simulink model "commtimrecresample"  (Simulink 7.2)
settings: Solver=ode45  StartTime=0.0  StopTime=5e-3  MaxStep=1/(10*D*Fsymbol)  RelTol=1e-3
PreLoadFcn:
  | Fsymbol=1e6;
  | D=8;  % decimation / interpolation
  | Fdelay = 5;  % rrc filter delay
  | Alpha = 0.25;  % excess BW
  | rrc_coef=rcosine(1,D,'fir/sqrt',Alpha,Fdelay);
  | rrc_coef=rrc_coef/sum(rrc_coef);
  | Carrier_Freq = 21.4e6;
  | b3 = [1/6 -1/2  1/2 -1/6];
  | b2 = [1/2 -1    1/2  0];
  | b1 = [1/3  1/2 -1    1/6];
  | b0 = [0    1    0    0];
undefined symbols (not defined in the file or in its folder): dfilt, j, magnitude
libraries: dspsigops x29, simulink x12, dsparch4 x8, commsynccomp2 x3, dspbuff3 x2, commblksprivate x1, dspmlti4 x1, commsink2 x1
Description:
  | Timing Recovery using Fixed-Rate Resampling
CloseFcn:
  | clear Fsymbol D Fdelay Alpha rrc_coef Carrier_Freq b0 b1 b2 b3;
settings Model: Creator=The MathWorks Inc.  LastModifiedBy=user
settings SolverCC: InsertRTBMode=Auto  SignalSizeVariationType=Allow to vary during execution
settings DataIOCC: SaveOutput=off  SignalLogging=off  SaveTime=off
settings OptimizationCC: InitFltsAndDblsToZero=on  EfficientMapNaN2IntZero=off
settings DebuggingCC: SaveWithParameterizedLinksMsg=none  SignalResolutionControl=TryResolveAllWithWarning  MultiTaskDSMMsg=warning  MultiTaskCondExecSysMsg=none  SigSpecEnsureSampleTimeMsg=none  StrictBusMsg=None
settings RTWCC: IncludeERTFirstTime=on
settings GRTTargetCC: TargetFcnLib=ansi_tfl_tmw.mat

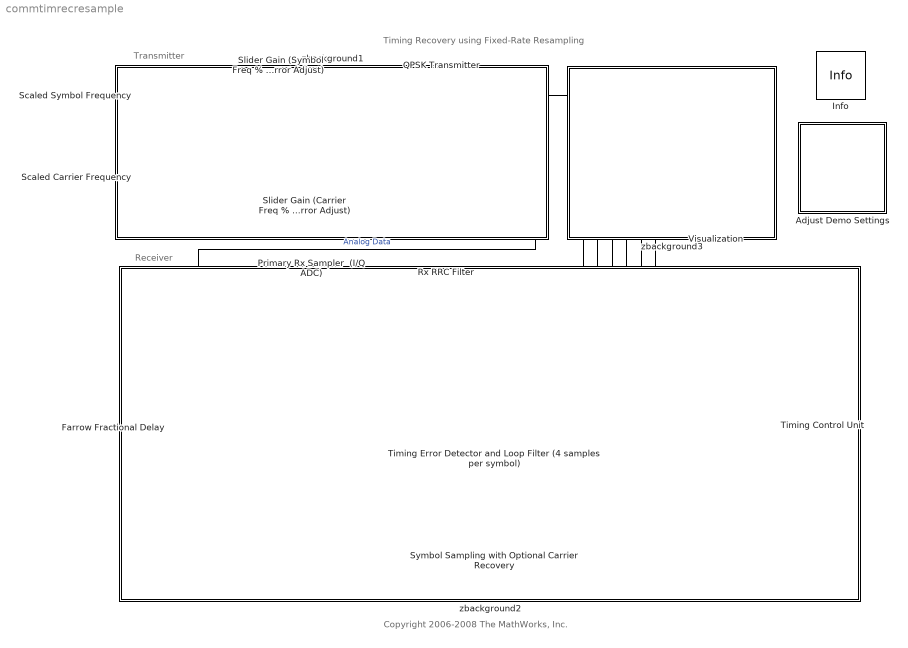
== system commtimrecresample ==
  note: Timing Recovery using Fixed-Rate Resampling
  note: Transmitter
  note: Receiver
  note: Copyright 2006-2008 The MathWorks, Inc.
  Adjust Demo Settings : Subsystem  mask(Timing Recovery Demo Settings){enableCarrierRec=on, enableTCU=on}
      mask prompts: enableCarrierRec "Enable carrier recovery"; enableTCU "Enable timing control"
      mask help:
      | Adjust these demo parameter settings to change the characteristics of the timing recovery (receiver) subsystem.  These settings may be changed while the demo is running.
      |
      | Note that you can also change the slider gain values for Symbol Frequency Percent Error and Carrier Frequency Percent Error while the demo is running.
      mask init:
      | set_param([bdroot(gcb) '/Symbol Sampling with Optional Carrier Recovery/Carrier_Rec_ON'],'Value',num2str(enableCarrierRec));
      | set_param([bdroot(gcb) '/Timing Control Unit/TCU_ON'],'Value',num2str(enableTCU));
      mask Help: helpview(commdhelp);
      mask Display: disp('Timing\nRecovery\nDemo\nSettings');
  "Farrow Fractional Delay " : Subsystem
  Info : commblksprivate/Info  SystemSampleTime=-1
  Primary Rx Sampler  (I/Q ADC) : ZeroOrderHold  SampleTime=1/(D*Fsymbol)
  QPSK Transmitter : Subsystem
  Rx RRC Filter : dspmlti4/FIR Decimation  DialogController=dspdialog.FIRDecimation  DialogControllerArgs=DataTag5  h=rrc_coef  D=2  filtStruct=Direct form  framing=Maintain input frame size  outputBufInitCond=0  roundingMode=Floor  overflowMode=off  FilterSource=Specify via dialog  FilterObject=Hm_firdecim
  Scaled Carrier Frequency : Constant  Value=Carrier_Freq / 100  OutDataType=sfix(16)  OutScaling=2^0
  Scaled Symbol Frequency : Constant  Value=(D*Fsymbol) / 100  OutDataType=sfix(16)  OutScaling=2^0
  Slider Gain (Carrier Freq % Error Adjust) : simulink/Math Operations/Slider Gain  SystemSampleTime=-1  low=-0.2  gain=-0.02  high=0.2
  Slider Gain (Symbol Freq % Error Adjust) : simulink/Math Operations/Slider Gain  SystemSampleTime=-1  low=-0.2  gain=0.05  high=0.2
  Symbol Sampling with Optional Carrier Recovery : Subsystem
  Timing Control Unit : Subsystem
  Timing Error Detector and Loop Filter (4 samples per symbol) : Subsystem
  Visualization : Subsystem
  zbackground1 : Subsystem
      mask Display: disp('')
  zbackground2 : Subsystem
      mask Display: disp('')
  zbackground3 : Subsystem
      mask Display: disp('')
  wires:
  Scaled Symbol Frequency/1 -> Slider Gain (Symbol Freq % Error Adjust)/1
  Slider Gain (Symbol Freq % Error Adjust)/1 -> QPSK Transmitter/1(Tx Sym Err)
  Slider Gain (Carrier Freq % Error Adjust)/1 -> QPSK Transmitter/2(Tx Car Err)
  Scaled Carrier Frequency/1 -> Slider Gain (Carrier Freq % Error Adjust)/1
  QPSK Transmitter/1(Tx Sym Clk) -> Visualization/1(Tx Sym Clk)
  QPSK Transmitter/2(Tx Data) -> Primary Rx Sampler  (I/Q ADC)/1  "Analog Data"
  "Farrow Fractional Delay "/1(X(n-(1-u))) -> Timing Error Detector and Loop Filter (4 samples per symbol)/2(I/Q In), Symbol Sampling with Optional Carrier Recovery/2(Data)
  Primary Rx Sampler  (I/Q ADC)/1 -> Rx RRC Filter/1
  Rx RRC Filter/1 -> "Farrow Fractional Delay "/1(X(n))
  Timing Control Unit/1(Symbol Clk) -> Timing Error Detector and Loop Filter (4 samples per symbol)/1(Symbol Clk), Symbol Sampling with Optional Carrier Recovery/1(Symbol Clk), Visualization/2(Rx Rec Sym Clk)
  Timing Control Unit/2(Delay Ctrl) -> "Farrow Fractional Delay "/2(u), Visualization/7(Frac Dly Ctrl)
  Timing Error Detector and Loop Filter (4 samples per symbol)/2(Timing Ctrl) -> Timing Control Unit/1(Ctrl In), Visualization/4(TCU Ctrl)
  Timing Error Detector and Loop Filter (4 samples per symbol)/1(Timing Err) -> Visualization/3(Timing Err)
  Symbol Sampling with Optional Carrier Recovery/1(Delayed Clk) -> Visualization/5(Delayed Clk)
  Symbol Sampling with Optional Carrier Recovery/2(Symbol) -> Visualization/6(Rx Symbol)

== system commtimrecresample/Adjust Demo Settings ==

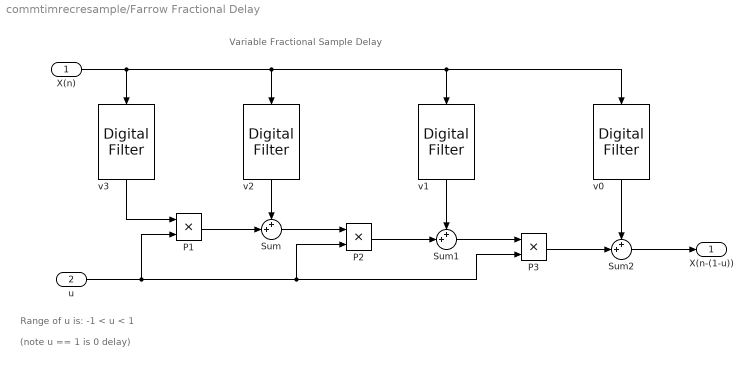
== system commtimrecresample/Farrow Fractional Delay  ==
  note: Range of u is: -1 < u < 1
  note: Variable Fractional Sample Delay
  note: (note u == 1 is 0 delay)
  X(n) : Inport  OutDataType=sfix(16)  OutScaling=2^0
  u : Inport  Port=2  OutDataType=sfix(16)  OutScaling=2^0
  P1 : Product  OutDataType=sfix(16)  OutScaling=2^0  SaturateOnIntegerOverflow=on  OutDataTypeStr=Inherit: Same as first input
  P2 : Product  OutDataType=sfix(16)  OutScaling=2^0  SaturateOnIntegerOverflow=on  OutDataTypeStr=Inherit: Same as first input
  P3 : Product  OutDataType=sfix(16)  OutScaling=2^0  SaturateOnIntegerOverflow=on  OutDataTypeStr=Inherit: Same as first input
  Sum : Sum  Inputs=++|  OutDataType=sfix(16)  OutScaling=2^0  SaturateOnIntegerOverflow=on
  Sum1 : Sum  Inputs=++|  OutDataType=sfix(16)  OutScaling=2^0  SaturateOnIntegerOverflow=on
  Sum2 : Sum  Inputs=++|  OutDataType=sfix(16)  OutScaling=2^0  SaturateOnIntegerOverflow=on
  v0 : dsparch4/Digital Filter  Orientation=down  DialogController=dspdialog.DigitalFilter  DialogControllerArgs=DataTag0  TypePopup=FIR (all zeros)  IIRFiltStruct=Direct form II transposed  AllPoleFiltStruct=Direct form  FIRFiltStruct=Direct form  CoeffSource=Specify via dialog  NumCoeffs=b0  DenCoeffs=[1 0.1]  BiQuadCoeffs=[1 0.3 0.4 1 0.1 0.2]  LatticeCoeffs=[0.2 0.4]  denIgnore=on  FiltPerSampPopup=One filter per frame  IC=0  ICnum=0  ICden=0  roundingMode=Floor  overflowMode=off  ScaleValues=1  scaleValueFracLength=14  stageInFracLength=15  stageOutFracLength=15  FilterSource=Specify via dialog  dfiltObjectName=dfilt.dffir([1 2 1])
  v1 : dsparch4/Digital Filter  Orientation=down  DialogController=dspdialog.DigitalFilter  DialogControllerArgs=DataTag1  TypePopup=FIR (all zeros)  IIRFiltStruct=Direct form II transposed  AllPoleFiltStruct=Direct form  FIRFiltStruct=Direct form  CoeffSource=Specify via dialog  NumCoeffs=b1  DenCoeffs=[1 0.1]  BiQuadCoeffs=[1 0.3 0.4 1 0.1 0.2]  LatticeCoeffs=[0.2 0.4]  denIgnore=on  FiltPerSampPopup=One filter per frame  IC=0  ICnum=0  ICden=0  roundingMode=Floor  overflowMode=off  ScaleValues=1  scaleValueFracLength=14  stageInFracLength=15  stageOutFracLength=15  FilterSource=Specify via dialog  dfiltObjectName=dfilt.dffir([1 2 1])
  v2 : dsparch4/Digital Filter  Orientation=down  DialogController=dspdialog.DigitalFilter  DialogControllerArgs=DataTag2  TypePopup=FIR (all zeros)  IIRFiltStruct=Direct form II transposed  AllPoleFiltStruct=Direct form  FIRFiltStruct=Direct form  CoeffSource=Specify via dialog  NumCoeffs=b2  DenCoeffs=[1 0.1]  BiQuadCoeffs=[1 0.3 0.4 1 0.1 0.2]  LatticeCoeffs=[0.2 0.4]  denIgnore=on  FiltPerSampPopup=One filter per frame  IC=0  ICnum=0  ICden=0  roundingMode=Floor  overflowMode=off  ScaleValues=1  scaleValueFracLength=14  stageInFracLength=15  stageOutFracLength=15  FilterSource=Specify via dialog  dfiltObjectName=dfilt.dffir([1 2 1])
  v3 : dsparch4/Digital Filter  Orientation=down  DialogController=dspdialog.DigitalFilter  DialogControllerArgs=DataTag3  TypePopup=FIR (all zeros)  IIRFiltStruct=Direct form II transposed  AllPoleFiltStruct=Direct form  FIRFiltStruct=Direct form  CoeffSource=Specify via dialog  NumCoeffs=b3  DenCoeffs=[1 0.1]  BiQuadCoeffs=[1 0.3 0.4 1 0.1 0.2]  LatticeCoeffs=[0.2 0.4]  denIgnore=on  FiltPerSampPopup=One filter per frame  IC=0  ICnum=0  ICden=0  roundingMode=Floor  overflowMode=off  ScaleValues=1  scaleValueFracLength=14  stageInFracLength=15  stageOutFracLength=15  FilterSource=Specify via dialog  dfiltObjectName=dfilt.dffir([1 2 1])
  X(n-(1-u)) : Outport  OutDataType=sfix(16)  OutScaling=2^0
  wires:
  Sum2/1 -> X(n-(1-u))/1
  u/1 -> P3/2, P2/2, P1/2
  X(n)/1 -> v3/1, v2/1, v1/1, v0/1
  v0/1 -> Sum2/1
  v1/1 -> Sum1/1
  v2/1 -> Sum/1
  v3/1 -> P1/1
  P1/1 -> Sum/2
  Sum/1 -> P2/1
  P2/1 -> Sum1/2
  Sum1/1 -> P3/1
  P3/1 -> Sum2/2

== system commtimrecresample/QPSK Transmitter ==
  note: 1/Ts=D*Fsymbol
  Tx Sym Err : Inport  OutDataType=sfix(16)  OutScaling=2^0
  Tx Car Err : Inport  Port=2  OutDataType=sfix(16)  OutScaling=2^0
  Carrier Offset and Conversion to Continuous Time : Subsystem
  Variable Rate Symbol Generator : Subsystem  TreatAsAtomicUnit=on
  Voltage-Controlled Oscillator : commsynccomp2/Continuous-Time VCO  SystemSampleTime=-1  Ac=1  Fc=D*Fsymbol  Kc=1  Ph=pi
  Tx Sym Clk : Outport  OutDataType=sfix(16)  OutScaling=2^0
  Tx Data : Outport  Port=2  OutDataType=sfix(16)  OutScaling=2^0
  wires:
  Variable Rate Symbol Generator/1(RRC'd Symbols) -> Carrier Offset and Conversion to Continuous Time/1(Data)
  Voltage-Controlled Oscillator/1 -> Variable Rate Symbol Generator/Trigger
  Carrier Offset and Conversion to Continuous Time/1(I/Q Out) -> Tx Data/1  "Baseband Continuous-Time Data"
  Tx Car Err/1 -> Carrier Offset and Conversion to Continuous Time/2(Error)
  Tx Sym Err/1 -> Voltage-Controlled Oscillator/1
  Variable Rate Symbol Generator/2(Symbol Clk) -> Tx Sym Clk/1  "Symbol Clock"

== system commtimrecresample/Symbol Sampling with Optional Carrier Recovery ==
  note: Subsequent processing (demodulation, error correction, symbol to bit mapping, etc.)
      | may be placed inside the Symbol Sampler block.
  Symbol Clk : Inport  OutDataType=sfix(16)  OutScaling=2^0
  Data : Inport  Port=2  OutDataType=sfix(16)  OutScaling=2^0
  Carrier_Rec_ON : Constant  OutDataTypeMode=boolean  OutDataType=sfix(16)  OutScaling=2^0  OutDataTypeStr=boolean
  Delay : dspsigops/Delay  dly_unit=Samples  delay=2  ic_detail=off  dif_ic_for_ch=off  dif_ic_for_dly=off  ic=0  reset_popup=None
  Symbol Sampler : Subsystem  TreatAsAtomicUnit=on
  Delayed Clk : Outport  OutDataType=sfix(16)  OutScaling=2^0
  Symbol : Outport  Port=2  OutDataType=sfix(16)  OutScaling=2^0
  wires:
  Delay/1 -> Delayed Clk/1, Symbol Sampler/Enable
  Symbol Clk/1 -> Delay/1
  Data/1 -> Symbol Sampler/1(In1)
  Symbol Sampler/1(Out1) -> Symbol/1
  Carrier_Rec_ON/1 -> Symbol Sampler/2(Carrier Recovery ON)

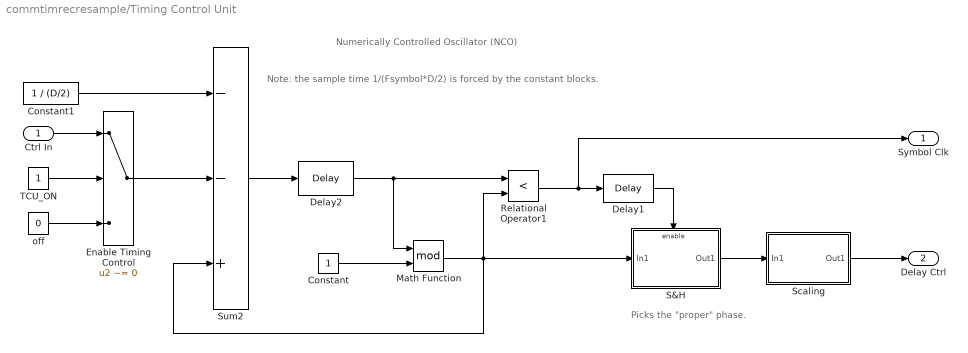
== system commtimrecresample/Timing Control Unit ==
  note: Note:  the sample time 1/(Fsymbol*D/2)
      | is forced by the constant blocks.
  note: Numerically Controlled Oscillator (NCO)
  note: Picks the "proper" phase.
  Ctrl In : Inport  OutDataType=sfix(16)  OutScaling=2^0
  Constant : Constant  OutDataType=sfix(16)  OutScaling=2^0  OutDataTypeStr=Inherit: Inherit via back propagation  SampleTime=1/(Fsymbol*D/2)
  Constant1 : Constant  Value=1 / (D/2)  OutDataType=sfix(16)  OutScaling=2^0  OutDataTypeStr=Inherit: Inherit via back propagation  SampleTime=1/(Fsymbol*D/2)
  Delay1 : dspsigops/Delay  dly_unit=Samples  delay=1  ic_detail=off  dif_ic_for_ch=off  dif_ic_for_dly=off  ic=0  reset_popup=None
  Delay2 : dspsigops/Delay  dly_unit=Samples  delay=1  ic_detail=on  dif_ic_for_ch=off  dif_ic_for_dly=off  ic=0  reset_popup=None
  Enable Timing Control : Switch  Criteria=u2 ~= 0
  Math Function : Math  Operator=mod  OutDataType=sfix(16)  OutScaling=2^0  SaturateOnIntegerOverflow=on
  Relational Operator1 : RelationalOperator  Operator=<  LogicOutDataTypeMode=boolean  LogicDataType=double(64)  OutDataTypeStr=boolean
  "S&H " : Subsystem  TreatAsAtomicUnit=on
  Scaling : Subsystem
  Sum2 : Sum  Inputs=--+  OutDataType=sfix(16)  OutScaling=2^0  SaturateOnIntegerOverflow=on  InputSameDT=on  OutDataTypeStr=Inherit: Same as first input
  TCU_ON : Constant  OutDataTypeMode=boolean  OutDataType=sfix(16)  OutScaling=2^0  OutDataTypeStr=boolean
  off : Constant  Value=0  OutDataType=sfix(16)  OutScaling=2^0
  Symbol Clk : Outport  OutDataType=sfix(16)  OutScaling=2^0
  Delay Ctrl : Outport  Port=2  OutDataType=sfix(16)  OutScaling=2^0
  wires:
  Delay2/1 -> Math Function/1, Relational Operator1/1
  Constant/1 -> Math Function/2
  Sum2/1 -> Delay2/1
  Constant1/1 -> Sum2/1
  Math Function/1 -> Sum2/3, Relational Operator1/2, "S&H "/1(In1)
  Relational Operator1/1 -> Delay1/1, Symbol Clk/1
  Delay1/1 -> "S&H "/Enable
  "S&H "/1(Out1) -> Scaling/1(In1)
  Scaling/1(Out1) -> Delay Ctrl/1
  TCU_ON/1 -> Enable Timing Control/2
  off/1 -> Enable Timing Control/3
  Ctrl In/1 -> Enable Timing Control/1
  Enable Timing Control/1 -> Sum2/2

== system commtimrecresample/Timing Error Detector and Loop Filter (4 samples per symbol) ==
  note: H. Meyer et. al. Digital Communications Receivers, chapter 5.4, pp 291
  Symbol Clk : Inport  OutDataType=sfix(16)  OutScaling=2^0
  I/Q In : Inport  Port=2  OutDataType=sfix(16)  OutScaling=2^0
  Mag Sq + Delays : Subsystem
  Timing Error Detector : Subsystem  TreatAsAtomicUnit=on
  Timing Err : Outport  OutDataType=sfix(16)  OutScaling=2^0
  Timing Ctrl : Outport  Port=2  OutDataType=sfix(16)  OutScaling=2^0
  wires:
  Mag Sq + Delays/1(MagSq(u[n-1])) -> Timing Error Detector/1(In1)
  Mag Sq + Delays/2(MagSq(u[n-3])) -> Timing Error Detector/2(In2)
  Mag Sq + Delays/3(MagSq(u[n-2])) -> Timing Error Detector/3(In3)
  Mag Sq + Delays/4(MagSq(u[n])) -> Timing Error Detector/4(In4)
  I/Q In/1 -> Mag Sq + Delays/1(In1)
  Timing Error Detector/1(Error) -> Timing Err/1
  Timing Error Detector/2(Cntrl) -> Timing Ctrl/1
  Symbol Clk/1 -> Timing Error Detector/Enable

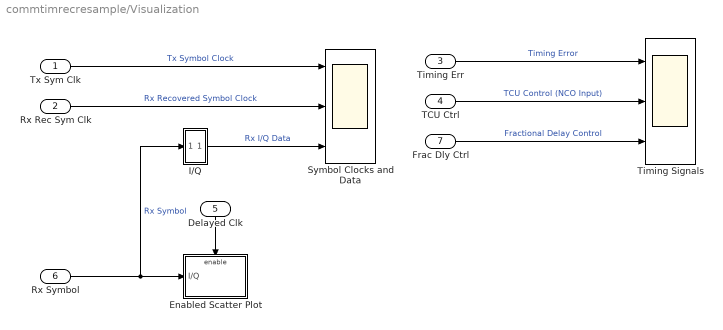
== system commtimrecresample/Visualization ==
  Tx Sym Clk : Inport  OutDataType=sfix(16)  OutScaling=2^0
  Rx Rec Sym Clk : Inport  Port=2  OutDataType=sfix(16)  OutScaling=2^0
  Timing Err : Inport  Port=3  OutDataType=sfix(16)  OutScaling=2^0
  TCU Ctrl : Inport  Port=4  OutDataType=sfix(16)  OutScaling=2^0
  Delayed Clk : Inport  Orientation=down  Port=5  OutDataType=sfix(16)  OutScaling=2^0
  Rx Symbol : Inport  Port=6  OutDataType=sfix(16)  OutScaling=2^0
  Frac Dly Ctrl : Inport  Port=7  OutDataType=sfix(16)  OutScaling=2^0
  Enabled Scatter Plot : Subsystem  TreatAsAtomicUnit=on
  I/Q : Subsystem
      mask Display: disp('')
  Symbol Clocks and Data : Scope  NumInputPorts=3
      settings: TimeRange=2e-006  YMin=-0.1~-0.1~-1.5  YMax=1.1~1.1~1.5
  Timing Signals : Scope  NumInputPorts=3
      settings: TimeRange=0.0002  YMin=-0.2~-0.001~-0.1  YMax=0.2~0.001~1.1  MaxDataPoints=50000
  wires:
  Rx Symbol/1 -> I/Q/1(cmplx), Enabled Scatter Plot/1(I/Q)  "Rx Symbol"
  I/Q/1(2x real) -> Symbol Clocks and Data/3  "Rx I/Q Data"
  Tx Sym Clk/1 -> Symbol Clocks and Data/1  "Tx Symbol Clock"
  Rx Rec Sym Clk/1 -> Symbol Clocks and Data/2  "Rx Recovered Symbol Clock"
  Timing Err/1 -> Timing Signals/1  "Timing Error"
  TCU Ctrl/1 -> Timing Signals/2  "TCU Control (NCO Input)"
  Frac Dly Ctrl/1 -> Timing Signals/3  "Fractional Delay Control"
  Delayed Clk/1 -> Enabled Scatter Plot/Enable

== system commtimrecresample/zbackground1 ==

== system commtimrecresample/zbackground2 ==

== system commtimrecresample/zbackground3 ==

== system commtimrecresample/QPSK Transmitter/Carrier Offset and Conversion to Continuous Time ==
  Data : Inport  OutDataType=sfix(16)  OutScaling=2^0
  Error : Inport  Port=2  OutDataType=sfix(16)  OutScaling=2^0
  Bessel LPF : Subsystem
  Product : Product  OutDataType=sfix(16)  OutScaling=2^0  RndMeth=Zero
  Real-Imag to Complex : RealImagToComplex
  Voltage-Controlled Oscillator : commsynccomp2/Continuous-Time VCO  SystemSampleTime=-1  Ac=1  Fc=0  Kc=1  Ph=0
  Voltage-Controlled Oscillator1 : commsynccomp2/Continuous-Time VCO  SystemSampleTime=-1  Ac=1  Fc=0  Kc=1  Ph=-pi/2
  I/Q Out : Outport  OutDataType=sfix(16)  OutScaling=2^0
  wires:
  Voltage-Controlled Oscillator/1 -> Real-Imag to Complex/1
  Voltage-Controlled Oscillator1/1 -> Real-Imag to Complex/2
  Real-Imag to Complex/1 -> Product/2
  Data/1 -> Product/1
  Error/1 -> Voltage-Controlled Oscillator/1, Voltage-Controlled Oscillator1/1
  Product/1 -> Bessel LPF/1(In1)
  Bessel LPF/1(Out1) -> I/Q Out/1

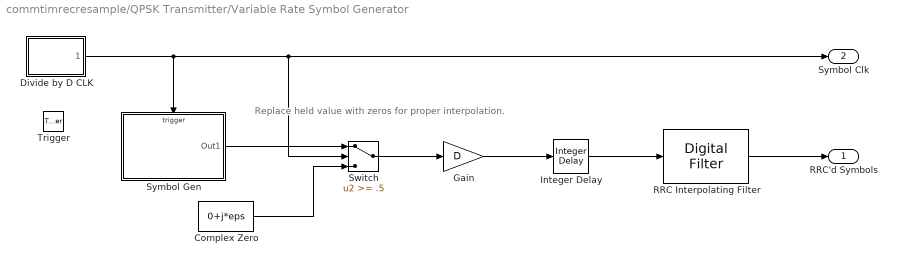
== system commtimrecresample/QPSK Transmitter/Variable Rate Symbol Generator ==
  note: Replace held value
      |  with zeros
      |  for proper interpolation.
  Trigger : TriggerPort
  Complex Zero : Constant  Value=0+j*eps  OutDataType=sfix(16)  OutScaling=2^0
  Divide by D CLK : Subsystem  TreatAsAtomicUnit=on  mask(Pulse Divider){div=D, ph=2}
      mask prompts: div "Modulo:"; ph "Initial Phase Delay (cycles):"
  Gain : Gain  Gain=D  ParameterDataType=sfix(16)  ParameterScaling=2^0  OutDataType=sfix(16)  OutScaling=2^0
  Integer Delay : simulink/Discrete/Integer Delay  vinit=0.0  samptime=-1  NumDelays=6
  RRC Interpolating Filter : dsparch4/Digital Filter  DialogController=dspdialog.DigitalFilter  DialogControllerArgs=DataTag4  TypePopup=FIR (all zeros)  IIRFiltStruct=Direct form II transposed  AllPoleFiltStruct=Direct form  FIRFiltStruct=Direct form  CoeffSource=Specify via dialog  NumCoeffs=rrc_coef  DenCoeffs=[1 0.1]  BiQuadCoeffs=[1 0.3 0.4 1 0.1 0.2]  LatticeCoeffs=[0.2 0.4]  denIgnore=on  FiltPerSampPopup=One filter per frame  IC=0  ICnum=0  ICden=0  roundingMode=Floor  overflowMode=off  ScaleValues=1  scaleValueFracLength=14  stageInFracLength=15  stageOutFracLength=15  FilterSource=Specify via dialog  dfiltObjectName=dfilt.dffir([1 2 1])
  Switch : Switch  Threshold=.5
  Symbol Gen : Subsystem  TreatAsAtomicUnit=on
  RRC'd Symbols : Outport  OutDataType=sfix(16)  OutScaling=2^0
  Symbol Clk : Outport  Port=2  OutDataType=sfix(16)  OutScaling=2^0
  wires:
  Divide by D CLK/1(" ") -> Symbol Gen/Trigger, Switch/2, Symbol Clk/1
  Symbol Gen/1(Out1) -> Switch/1
  Complex Zero/1 -> Switch/3
  Gain/1 -> Integer Delay/1
  RRC Interpolating Filter/1 -> RRC'd Symbols/1
  Switch/1 -> Gain/1
  Integer Delay/1 -> RRC Interpolating Filter/1

== system commtimrecresample/Symbol Sampling with Optional Carrier Recovery/Symbol Sampler ==
  In1 : Inport  OutDataType=sfix(16)  OutScaling=2^0
  Carrier Recovery ON : Inport  Port=2  OutDataType=sfix(16)  OutScaling=2^0
  Enable : EnablePort
  Carrier Recovery : Subsystem  TreatAsAtomicUnit=on
  Switch : Switch  Threshold=.5
  Out1 : Outport  OutDataType=sfix(16)  OutScaling=2^0  OutputWhenDisabled=reset  InitialOutput=0
  wires:
  Carrier Recovery ON/1 -> Carrier Recovery/Enable, Switch/2
  In1/1 -> Carrier Recovery/1(I/Q In), Switch/3
  Switch/1 -> Out1/1
  Carrier Recovery/1(Derotated I/Q Out) -> Switch/1

== system commtimrecresample/Timing Control Unit/S&H  ==
  In1 : Inport  OutDataType=sfix(16)  OutScaling=2^0
  Enable : EnablePort
  Out1 : Outport  OutDataType=sfix(16)  OutScaling=2^0
  wires:
  In1/1 -> Out1/1

== system commtimrecresample/Timing Control Unit/Scaling ==
  note: maps phase ramp of 0.5 to 0.75 to output of 0 to 1
  In1 : Inport  OutDataType=sfix(16)  OutScaling=2^0
  Add : Sum  OutDataType=sfix(16)  OutScaling=2^-10
  Gain2 : Gain  Gain=4  ParameterDataType=sfix(16)  ParameterScaling=2^0  OutDataType=sfix(16)  OutScaling=2^0
  k5 : Constant  Value=-2  OutDataType=sfix(16)  OutScaling=2^0  SampleTime=1/(Fsymbol*D/2)
  Out1 : Outport  OutDataType=sfix(16)  OutScaling=2^0
  wires:
  Add/1 -> Out1/1
  In1/1 -> Gain2/1
  k5/1 -> Add/2
  Gain2/1 -> Add/1

== system commtimrecresample/Timing Error Detector and Loop Filter (4 samples per symbol)/Mag Sq + Delays ==
  note: Taking the mag squared makes this symbol timing detector impervious to carrier frequency shift.
      | Therefore, the simpler job of carrier recovery can be done after symbol retiming.
  In1 : Inport  OutDataType=sfix(16)  OutScaling=2^0
  Delay1 : dspsigops/Delay  dly_unit=Samples  delay=1  ic_detail=off  dif_ic_for_ch=off  dif_ic_for_dly=off  ic=0  reset_popup=None
  Delay2 : dspsigops/Delay  dly_unit=Samples  delay=1  ic_detail=off  dif_ic_for_ch=off  dif_ic_for_dly=off  ic=0  reset_popup=None
  Delay3 : dspsigops/Delay  dly_unit=Samples  delay=1  ic_detail=off  dif_ic_for_ch=off  dif_ic_for_dly=off  ic=0  reset_popup=None
  Math Function : Math  Operator=magnitude^2  OutDataType=sfix(16)  OutScaling=2^0  SaturateOnIntegerOverflow=on
  MagSq(u[n-1]) : Outport  OutDataType=sfix(16)  OutScaling=2^0
  MagSq(u[n-3]) : Outport  Port=2  OutDataType=sfix(16)  OutScaling=2^0
  MagSq(u[n-2]) : Outport  Port=3  OutDataType=sfix(16)  OutScaling=2^0
  MagSq(u[n]) : Outport  Port=4  OutDataType=sfix(16)  OutScaling=2^0
  wires:
  In1/1 -> Math Function/1
  Math Function/1 -> Delay1/1, MagSq(u[n])/1
  Delay1/1 -> Delay2/1, MagSq(u[n-1])/1
  Delay2/1 -> Delay3/1, MagSq(u[n-2])/1
  Delay3/1 -> MagSq(u[n-3])/1

== system commtimrecresample/Timing Error Detector and Loop Filter (4 samples per symbol)/Timing Error Detector ==
  note: update once per symbol
  note: 4 samples per symbol are required
      | for this timing error estimator.
  In1 : Inport  OutDataType=sfix(16)  OutScaling=2^0
  In2 : Inport  Port=2  OutDataType=sfix(16)  OutScaling=2^0
  In3 : Inport  Port=3  OutDataType=sfix(16)  OutScaling=2^0
  In4 : Inport  Port=4  OutDataType=sfix(16)  OutScaling=2^0
  Enable : EnablePort
  "Loop Filter " : Subsystem  TreatAsAtomicUnit=on
  Timing Error : Subsystem
  Error : Outport  OutDataType=sfix(16)  OutScaling=2^0
  Cntrl : Outport  Port=2  OutDataType=sfix(16)  OutScaling=2^0
  wires:
  Timing Error/1(Out1) -> "Loop Filter "/1(In1), Error/1
  In1/1 -> Timing Error/1(In1)
  In2/1 -> Timing Error/2(In2)
  In3/1 -> Timing Error/3(In3)
  In4/1 -> Timing Error/4(In4)
  "Loop Filter "/1(Out1) -> Cntrl/1

== system commtimrecresample/Visualization/Enabled Scatter Plot ==
  note: You can add demodulator, FEC, etc.
      | in this enabled subsystem.
  I/Q : Inport  OutDataType=sfix(16)  OutScaling=2^0
  Enable : EnablePort
  Discrete-Time Scatter Plot Scope2 : commsink2/Discrete-Time Scatter Plot Scope  Tag=ScatterPlot  SystemSampleTime=-1  sampPerSymb=1  offsetEye=0  numTraces=31  numNewFrames=1  LineMarkers=.  LineColors=b  fading=off  render=on  AxisGrid=on  xMin=-2  xMax=2  yMin=-2  yMax=2  inphaseLabel=In-phase Amplitude  quadratureLabel=Quadrature Amplitude  openScopeAtSimStart=on  FrameNumber=off  FigPos=[650 336 317 317]  figTitle=Received Symbol  numLinesMax=8  block_type_=scatter
  wires:
  I/Q/1 -> Discrete-Time Scatter Plot Scope2/1

== system commtimrecresample/Visualization/I/Q ==
  note: to visually align traces
  cmplx : Inport  OutDataType=sfix(16)  OutScaling=2^0
  Complex to Real-Imag : ComplexToRealImag
  Delay1 : dspsigops/Delay  dly_unit=Samples  delay=2  ic_detail=off  dif_ic_for_ch=off  dif_ic_for_dly=off  ic=0  reset_popup=None
  Mux : Mux  Inputs=2
  2x real : Outport  OutDataType=sfix(16)  OutScaling=2^0
  wires:
  Complex to Real-Imag/1 -> Mux/1
  Complex to Real-Imag/2 -> Mux/2
  cmplx/1 -> Complex to Real-Imag/1
  Mux/1 -> Delay1/1
  Delay1/1 -> 2x real/1

== system commtimrecresample/QPSK Transmitter/Carrier Offset and Conversion to Continuous Time/Bessel LPF ==
  In1 : Inport  OutDataType=sfix(16)  OutScaling=2^0
  Analog Filter Design : dsparch4/Analog Filter Design  method=Bessel  filttype=Lowpass  N=8  Wlo=2*pi*D*Fsymbol*0.3  Whi=80  Rp=2  Rs=40
  Analog Filter Design1 : dsparch4/Analog Filter Design  method=Bessel  filttype=Lowpass  N=8  Wlo=2*pi*D*Fsymbol*0.3  Whi=80  Rp=2  Rs=40
  Complex to Real-Imag : ComplexToRealImag
  Real-Imag to Complex1 : RealImagToComplex
  Out1 : Outport  OutDataType=sfix(16)  OutScaling=2^0
  wires:
  Complex to Real-Imag/1 -> Analog Filter Design/1
  Complex to Real-Imag/2 -> Analog Filter Design1/1
  Analog Filter Design/1 -> Real-Imag to Complex1/1
  Analog Filter Design1/1 -> Real-Imag to Complex1/2
  Real-Imag to Complex1/1 -> Out1/1
  In1/1 -> Complex to Real-Imag/1

== system commtimrecresample/QPSK Transmitter/Variable Rate Symbol Generator/Divide by D CLK ==
  Constant1 : Constant  Orientation=up  Value=div  OutDataType=sfix(16)  OutScaling=2^0
  Constant2 : Constant  OutDataType=sfix(16)  OutScaling=2^0
  Fcn4 : Fcn  Expr=u<1
  Math Function : Math  Operator=mod  OutDataType=sfix(16)  OutScaling=2^0  SaturateOnIntegerOverflow=on
  Sum : Sum  Inputs=|++  OutDataType=sfix(16)  OutScaling=2^0  SaturateOnIntegerOverflow=on  InputSameDT=on  OutDataTypeStr=Inherit: Same as first input
  Unit Delay : UnitDelay  X0=div-ph  SampleTime=-1
  " " : Outport  OutDataType=sfix(16)  OutScaling=2^0
  wires:
  Fcn4/1 -> " "/1
  Constant1/1 -> Math Function/2
  Math Function/1 -> Fcn4/1, Sum/2
  Unit Delay/1 -> Math Function/1
  Constant2/1 -> Sum/1
  Sum/1 -> Unit Delay/1

== system commtimrecresample/QPSK Transmitter/Variable Rate Symbol Generator/Symbol Gen ==
  Trigger : TriggerPort
  PN1 : Subsystem  AncestorBlock=RF/GPS Blocks/C//A Code, 1.023MHz/PN1  mask(PN(10) Sequence [3,10]){}
      mask help: Pseudo Noise Sequence (M=2^10 - 1, Feedback[3,10])
      mask init:
      | [x,y]=commsrcsicon(5);
      mask Help: Maximal length pseudo-noise sequence with 10 memory elements.  Feedback is from taps 3 and 10.  Only the 10th tap is output.
      mask Display: plot(0,0,100,100,x,y);disp('PN Sequence ')
  QPSK : Subsystem
  Out1 : Outport  OutDataType=sfix(16)  OutScaling=2^0
  wires:
  PN1/1(Tap10) -> QPSK/1(In1)
  PN1/2(Tap2) -> QPSK/2(In2)
  QPSK/1(Out1) -> Out1/1

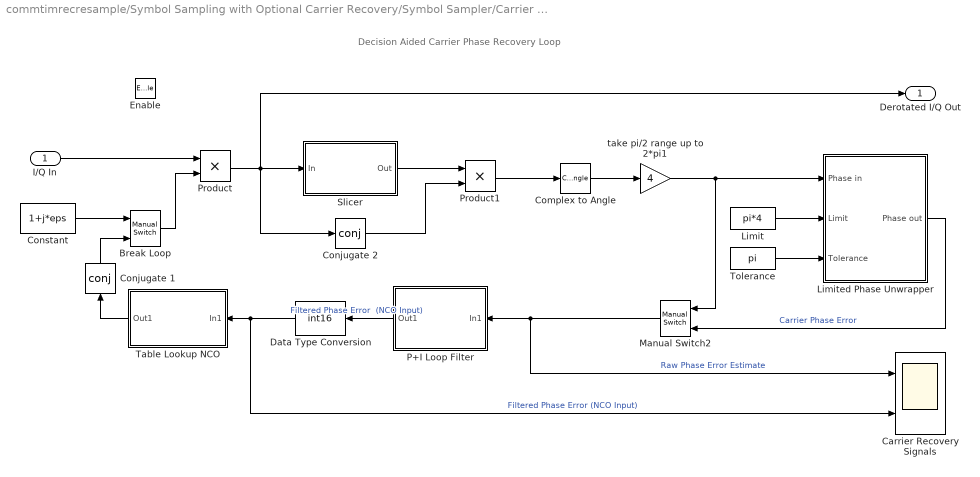
== system commtimrecresample/Symbol Sampling with Optional Carrier Recovery/Symbol Sampler/Carrier Recovery ==
  note: Decision Aided Carrier Phase Recovery Loop
  I/Q In : Inport  OutDataType=sfix(16)  OutScaling=2^0
  Enable : EnablePort
  Break Loop : simulink/Signal Routing/Manual Switch  SystemSampleTime=-1  sw=0  action=0  varsize=off
  Carrier Recovery Signals : Scope  NumInputPorts=2
      settings: TimeRange=0.0002  YMin=-0.5~-10  YMax=0.5~10  SaveName=ScopeData2  MaxDataPoints=50000
  Complex to Angle : ComplexToMagnitudeAngle  Output=Angle
  Conjugate 1 : Math  Orientation=up  Operator=conj  OutDataType=sfix(16)  OutScaling=2^0  SaturateOnIntegerOverflow=on
  Conjugate 2 : Math  Operator=conj  OutDataType=sfix(16)  OutScaling=2^0  SaturateOnIntegerOverflow=on
  Constant : Constant  Value=1+j*eps  OutDataType=sfix(16)  OutScaling=2^0
  Data Type Conversion : DataTypeConversion  Orientation=left  OutDataTypeMode=int16  OutDataType=sfix(16)  OutScaling=2^0  OutDataTypeStr=int16  RndMeth=Nearest  SaturateOnIntegerOverflow=on
  Limit : Constant  Value=pi*4  VectorParams1D=off  OutDataType=sfix(16)  OutScaling=2^0
  Limited Phase Unwrapper : Subsystem
  Manual Switch2 : simulink/Signal Routing/Manual Switch  Orientation=left  SystemSampleTime=-1  sw=0  action=0  varsize=off
  P+I Loop Filter : Subsystem  Orientation=left
  Product : Product  OutDataType=sfix(16)  OutScaling=2^0  RndMeth=Zero
  Product1 : Product  OutDataType=sfix(16)  OutScaling=2^0  RndMeth=Zero
  Slicer : Subsystem
  Table Lookup NCO : Subsystem  Orientation=left
  Tolerance : Constant  Value=pi  VectorParams1D=off  OutDataType=sfix(16)  OutScaling=2^0
  take pi/2 range up to 2*pi1 : Gain  Gain=4  ParameterDataType=sfix(16)  ParameterScaling=2^0  OutDataType=sfix(16)  OutScaling=2^0
  Derotated I/Q Out : Outport  OutDataType=sfix(16)  OutScaling=2^0
  wires:
  P+I Loop Filter/1(Out1) -> Data Type Conversion/1  "Filtered Phase Error  (NCO Input)"
  Table Lookup NCO/1(Out1) -> Conjugate 1/1
  Constant/1 -> Break Loop/1
  Conjugate 1/1 -> Break Loop/2
  Break Loop/1 -> Product/2
  Product1/1 -> Complex to Angle/1
  Conjugate 2/1 -> Product1/2
  Slicer/1(Out) -> Product1/1
  Product/1 -> Derotated I/Q Out/1, Conjugate 2/1, Slicer/1(In)
  I/Q In/1 -> Product/1
  Complex to Angle/1 -> take pi/2 range up to 2*pi1/1
  Limit/1 -> Limited Phase Unwrapper/2(Limit)
  Tolerance/1 -> Limited Phase Unwrapper/3(Tolerance)
  Limited Phase Unwrapper/1(Phase out) -> Manual Switch2/2  "Carrier Phase Error"
  Manual Switch2/1 -> P+I Loop Filter/1(In1), Carrier Recovery Signals/1  "Raw Phase Error Estimate"
  take pi/2 range up to 2*pi1/1 -> Limited Phase Unwrapper/1(Phase in), Manual Switch2/1
  Data Type Conversion/1 -> Table Lookup NCO/1(In1), Carrier Recovery Signals/2  "Filtered Phase Error (NCO Input)"

== system commtimrecresample/Timing Error Detector and Loop Filter (4 samples per symbol)/Timing Error Detector/Loop Filter  ==
  note: Integrator
  note: PID Loop Filter
  In1 : Inport  OutDataType=sfix(16)  OutScaling=2^0
  Derivative : Gain  Gain=10  ParameterDataType=sfix(16)  ParameterScaling=2^0  OutDataType=sfix(16)  OutScaling=2^0
  Digital Filter : dsparch4/Digital Filter  DialogController=dspdialog.DigitalFilter  DialogControllerArgs=DataTag6  TypePopup=IIR (poles & zeros)  IIRFiltStruct=Direct form II transposed  AllPoleFiltStruct=Direct form  FIRFiltStruct=Direct form  CoeffSource=Specify via dialog  NumCoeffs=[.02]  DenCoeffs=[1 -1]  BiQuadCoeffs=[1 0.3 0.4 1 0.1 0.2]  LatticeCoeffs=[0.2 0.4]  denIgnore=on  FiltPerSampPopup=One filter per frame  IC=0  ICnum=0  ICden=0  roundingMode=Floor  overflowMode=off  ScaleValues=1  scaleValueFracLength=14  stageInFracLength=15  stageOutFracLength=15  FilterSource=Specify via dialog  dfiltObjectName=dfilt.dffir([1 2 1])
  Gain1 : Gain  Gain=-0.001  ParameterDataType=sfix(16)  ParameterScaling=2^0  OutDataType=sfix(16)  OutScaling=2^0
  Integer Delay : simulink/Discrete/Integer Delay  vinit=0.0  samptime=-1  NumDelays=5
  Proportional : Gain  Gain=5  ParameterDataType=sfix(16)  ParameterScaling=2^0  OutDataType=sfix(16)  OutScaling=2^0
  Smoothing Filter : DiscreteTransferFcn  Numerator=0.05  Denominator=[1 -0.95]  SampleTime=-1
  Sum1 : Sum  Inputs=+++  OutDataType=sfix(16)  OutScaling=2^0  SaturateOnIntegerOverflow=on  InputSameDT=on  OutDataTypeStr=Inherit: Same as first input
  Sum2 : Sum  Inputs=+-  OutDataType=sfix(16)  OutScaling=2^0  SaturateOnIntegerOverflow=on  InputSameDT=on  OutDataTypeStr=Inherit: Same as first input
  Out1 : Outport  OutDataType=sfix(16)  OutScaling=2^0
  wires:
  In1/1 -> Digital Filter/1, Smoothing Filter/1
  Digital Filter/1 -> Sum1/1
  Sum1/1 -> Gain1/1
  Integer Delay/1 -> Sum2/2
  Sum2/1 -> Derivative/1
  Proportional/1 -> Sum1/2
  Gain1/1 -> Out1/1
  Derivative/1 -> Sum1/3
  Smoothing Filter/1 -> Proportional/1, Integer Delay/1, Sum2/1

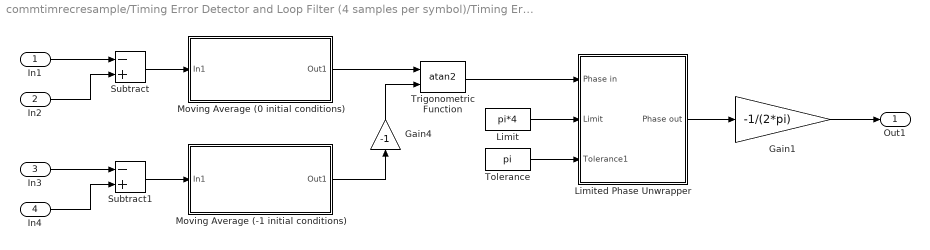
== system commtimrecresample/Timing Error Detector and Loop Filter (4 samples per symbol)/Timing Error Detector/Timing Error ==
  In1 : Inport  OutDataType=sfix(16)  OutScaling=2^0
  In2 : Inport  Port=2  OutDataType=sfix(16)  OutScaling=2^0
  In3 : Inport  Port=3  OutDataType=sfix(16)  OutScaling=2^0
  In4 : Inport  Port=4  OutDataType=sfix(16)  OutScaling=2^0
  Gain1 : Gain  Gain=-1/(2*pi)  ParameterDataType=sfix(16)  ParameterScaling=2^0  OutDataType=sfix(16)  OutScaling=2^0
  Gain4 : Gain  Orientation=up  Gain=-1  ParameterDataType=sfix(16)  ParameterScaling=2^0  OutDataType=sfix(16)  OutScaling=2^0
  Limit : Constant  Value=pi*4  VectorParams1D=off  OutDataType=sfix(16)  OutScaling=2^0
  Limited Phase Unwrapper : Subsystem
  Moving Average (-1 initial conditions) : Subsystem
  Moving Average (0 initial conditions) : Subsystem
  Subtract : Sum  Inputs=-+  OutDataType=sfix(16)  OutScaling=2^-10
  Subtract1 : Sum  Inputs=-+  OutDataType=sfix(16)  OutScaling=2^-10
  Tolerance : Constant  Value=pi  VectorParams1D=off  OutDataType=sfix(16)  OutScaling=2^0
  Trigonometric Function : Trigonometry  Operator=atan2
  Out1 : Outport  OutDataType=sfix(16)  OutScaling=2^0
  wires:
  In4/1 -> Subtract1/2
  In3/1 -> Subtract1/1
  In2/1 -> Subtract/2
  In1/1 -> Subtract/1
  Moving Average (-1 initial conditions)/1(Out1) -> Gain4/1
  Gain4/1 -> Trigonometric Function/2
  Limited Phase Unwrapper/1(Phase out) -> Gain1/1
  Gain1/1 -> Out1/1
  Subtract/1 -> Moving Average (0 initial conditions)/1(In1)
  Subtract1/1 -> Moving Average (-1 initial conditions)/1(In1)
  Trigonometric Function/1 -> Limited Phase Unwrapper/1(Phase in)
  Limit/1 -> Limited Phase Unwrapper/2(Limit)
  Tolerance/1 -> Limited Phase Unwrapper/3(Tolerance1)
  Moving Average (0 initial conditions)/1(Out1) -> Trigonometric Function/1

== system commtimrecresample/QPSK Transmitter/Variable Rate Symbol Generator/Symbol Gen/PN1 ==
  Subsystem : Subsystem
  Subsystem1 : Subsystem
  Terminator : Terminator
  Terminator1 : Terminator
  Tap10 : Outport  OutDataType=sfix(16)  OutScaling=2^0  InitialOutput=0
  Tap2 : Outport  Port=2  OutDataType=sfix(16)  OutScaling=2^0  InitialOutput=0
  wires:
  Subsystem/1(Tap10) -> Tap10/1
  Subsystem1/2(Tap2) -> Tap2/1
  Subsystem/2(Tap2) -> Terminator/1
  Subsystem1/1(Tap10) -> Terminator1/1

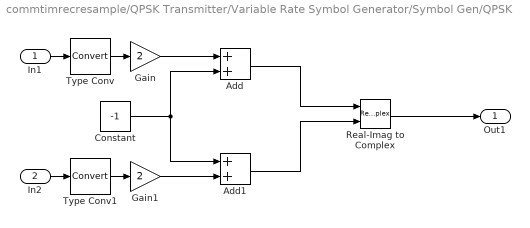
== system commtimrecresample/QPSK Transmitter/Variable Rate Symbol Generator/Symbol Gen/QPSK ==
  In1 : Inport  OutDataType=sfix(16)  OutScaling=2^0
  In2 : Inport  Port=2  OutDataType=sfix(16)  OutScaling=2^0
  Add : Sum  OutDataType=sfix(16)  OutScaling=2^-10
  Add1 : Sum  OutDataType=sfix(16)  OutScaling=2^-10
  Constant : Constant  Value=-1  OutDataType=sfix(16)  OutScaling=2^0
  Gain : Gain  Gain=2  ParameterDataType=sfix(16)  ParameterScaling=2^0  OutDataType=sfix(16)  OutScaling=2^0
  Gain1 : Gain  Gain=2  ParameterDataType=sfix(16)  ParameterScaling=2^0  OutDataType=sfix(16)  OutScaling=2^0
  Real-Imag to Complex : RealImagToComplex
  Type Conv : DataTypeConversion  OutDataType=sfix(16)  OutScaling=2^0
  Type Conv1 : DataTypeConversion  OutDataType=sfix(16)  OutScaling=2^0
  Out1 : Outport  OutDataType=sfix(16)  OutScaling=2^0
  wires:
  Real-Imag to Complex/1 -> Out1/1
  In2/1 -> Type Conv1/1
  Add/1 -> Real-Imag to Complex/1
  In1/1 -> Type Conv/1
  Gain/1 -> Add/1
  Constant/1 -> Add/2, Add1/1
  Gain1/1 -> Add1/2
  Add1/1 -> Real-Imag to Complex/2
  Type Conv/1 -> Gain/1
  Type Conv1/1 -> Gain1/1

== system commtimrecresample/Symbol Sampling with Optional Carrier Recovery/Symbol Sampler/Carrier Recovery/Limited Phase Unwrapper ==
  Phase in : Inport  OutDataType=sfix(16)  OutScaling=2^0
  Limit : Inport  Port=2  OutDataType=sfix(16)  OutScaling=2^0
  Tolerance : Inport  Port=3  OutDataType=sfix(16)  OutScaling=2^0
  Abs : Abs  SaturateOnIntegerOverflow=on
  Delay : dspsigops/Delay  dly_unit=Samples  delay=1  ic_detail=off  dif_ic_for_ch=off  dif_ic_for_dly=off  ic=0  reset_popup=None
  N*2*pi accumulator : Subsystem  TreatAsAtomicUnit=on
  Relational Operator : RelationalOperator
  Sum : Sum  Inputs=|-+  OutDataType=sfix(16)  OutScaling=2^0  SaturateOnIntegerOverflow=on
  Sum1 : Sum  Inputs=|++  OutDataType=sfix(16)  OutScaling=2^0  SaturateOnIntegerOverflow=on
  Phase out : Outport  OutDataType=sfix(16)  OutScaling=2^0
  wires:
  Phase in/1 -> Sum1/1, Sum/2, Delay/1
  Delay/1 -> Sum/1
  Sum/1 -> Abs/1, N*2*pi accumulator/1(add_sub)
  Abs/1 -> Relational Operator/1
  Tolerance/1 -> Relational Operator/2
  Relational Operator/1 -> N*2*pi accumulator/Enable
  N*2*pi accumulator/1(K*2*pi) -> Sum1/2
  Sum1/1 -> Phase out/1
  Limit/1 -> N*2*pi accumulator/2(Limit)

== system commtimrecresample/Symbol Sampling with Optional Carrier Recovery/Symbol Sampler/Carrier Recovery/P+I Loop Filter ==
  In1 : Inport  Orientation=left  OutDataType=sfix(16)  OutScaling=2^0
  Add : Sum  Orientation=left  OutDataType=sfix(16)  OutScaling=2^-10
  Add1 : Sum  Orientation=left  OutDataType=sfix(16)  OutScaling=2^-10
  I gain : Gain  Orientation=left  Gain=-.2  ParameterDataType=sfix(16)  ParameterScaling=2^0  OutDataType=sfix(16)  OutScaling=2^0
  Integer Delay : simulink/Discrete/Integer Delay  vinit=0.0  samptime=-1  NumDelays=1
  P gain : Gain  Orientation=left  Gain=-2  ParameterDataType=sfix(16)  ParameterScaling=2^0  OutDataType=sfix(16)  OutScaling=2^0
  Saturation : Saturate  UpperLimit=60  LowerLimit=-60
  Saturation1 : Saturate  Orientation=left  UpperLimit=60  LowerLimit=-60
  gain : Gain  Orientation=left  Gain=5  ParameterDataType=sfix(16)  ParameterScaling=2^0  OutDataType=sfix(16)  OutScaling=2^0
  Out1 : Outport  Orientation=left  OutDataType=sfix(16)  OutScaling=2^0
  wires:
  Add/1 -> Saturation1/1
  In1/1 -> gain/1
  I gain/1 -> Add1/1
  Integer Delay/1 -> Add1/2
  Add1/1 -> Add/2, Saturation/1
  P gain/1 -> Add/1
  gain/1 -> I gain/1, P gain/1
  Saturation/1 -> Integer Delay/1
  Saturation1/1 -> Out1/1

== system commtimrecresample/Symbol Sampling with Optional Carrier Recovery/Symbol Sampler/Carrier Recovery/Slicer ==
  In : Inport  OutDataType=sfix(16)  OutScaling=2^0
  Complex to Real-Imag : ComplexToRealImag
  Gain1 : Gain  Gain=1/sqrt(2)  ParameterDataType=sfix(16)  ParameterScaling=2^0  OutDataType=sfix(16)  OutScaling=2^0
  Real-Imag to Complex : RealImagToComplex
  Sign : Signum
  Sign1 : Signum
  Out : Outport  OutDataType=sfix(16)  OutScaling=2^0
  wires:
  In/1 -> Complex to Real-Imag/1
  Complex to Real-Imag/1 -> Sign/1
  Complex to Real-Imag/2 -> Sign1/1
  Sign/1 -> Real-Imag to Complex/1
  Sign1/1 -> Real-Imag to Complex/2
  Real-Imag to Complex/1 -> Gain1/1
  Gain1/1 -> Out/1

== system commtimrecresample/Symbol Sampling with Optional Carrier Recovery/Symbol Sampler/Carrier Recovery/Table Lookup NCO ==
  In1 : Inport  Orientation=left  OutDataType=sfix(16)  OutScaling=2^0
  Add2 : Sum  Orientation=left  OutDataType=sfix(16)  OutScaling=2^-10
  Constant1 : Constant  Value=(2^10)-1  OutDataType=sfix(16)  OutScaling=2^0
  Integer Delay1 : simulink/Discrete/Integer Delay  vinit=0.0  samptime=-1  NumDelays=1
  Math Function2 : Math  Orientation=left  Operator=mod  OutDataType=sfix(16)  OutScaling=2^0  SaturateOnIntegerOverflow=on
  Real-Imag to Complex : RealImagToComplex  Orientation=left
  cos : Lookup  Orientation=left  InputValues=[0:1023]  Table=cos((0:1023)*2*pi/1024)  LookUpMeth=Use Input Below  OutDataType=sfix(16)  OutScaling=2^0
  sin : Lookup  Orientation=left  InputValues=[0:1023]  Table=sin((0:1023)*2*pi/1024)  LookUpMeth=Use Input Below  OutDataType=sfix(16)  OutScaling=2^0
  Out1 : Outport  Orientation=left  OutDataType=sfix(16)  OutScaling=2^0
  wires:
  cos/1 -> Real-Imag to Complex/1
  sin/1 -> Real-Imag to Complex/2
  Math Function2/1 -> Integer Delay1/1
  Real-Imag to Complex/1 -> Out1/1
  In1/1 -> Add2/1
  Constant1/1 -> Math Function2/2
  Add2/1 -> Math Function2/1
  Integer Delay1/1 -> cos/1, sin/1, Add2/2

== system commtimrecresample/Timing Error Detector and Loop Filter (4 samples per symbol)/Timing Error Detector/Timing Error/Limited Phase Unwrapper ==
  Phase in : Inport  OutDataType=sfix(16)  OutScaling=2^0
  Limit : Inport  Port=2  OutDataType=sfix(16)  OutScaling=2^0
  Tolerance1 : Inport  Port=3  OutDataType=sfix(16)  OutScaling=2^0
  Abs : Abs  SaturateOnIntegerOverflow=on
  Delay : dspsigops/Delay  dly_unit=Samples  delay=1  ic_detail=off  dif_ic_for_ch=off  dif_ic_for_dly=off  ic=0  reset_popup=None
  N*2*pi accumulator : Subsystem  TreatAsAtomicUnit=on
  Relational Operator : RelationalOperator
  Sum : Sum  Inputs=|-+  OutDataType=sfix(16)  OutScaling=2^0  SaturateOnIntegerOverflow=on
  Sum1 : Sum  Inputs=|++  OutDataType=sfix(16)  OutScaling=2^0  SaturateOnIntegerOverflow=on
  Phase out : Outport  OutDataType=sfix(16)  OutScaling=2^0
  wires:
  Phase in/1 -> Sum1/1, Sum/2, Delay/1
  Delay/1 -> Sum/1
  Sum/1 -> Abs/1, N*2*pi accumulator/1(add_sub)
  Abs/1 -> Relational Operator/1
  Tolerance1/1 -> Relational Operator/2
  Relational Operator/1 -> N*2*pi accumulator/Enable
  N*2*pi accumulator/1(K*2*pi) -> Sum1/2
  Sum1/1 -> Phase out/1
  Limit/1 -> N*2*pi accumulator/2(Limit)

== system commtimrecresample/Timing Error Detector and Loop Filter (4 samples per symbol)/Timing Error Detector/Timing Error/Moving Average (-1 initial conditions) ==
  In1 : Inport  OutDataType=sfix(16)  OutScaling=2^0
  Delay Line1 : dspbuff3/Delay Line  siz=50  ic=-1  directfeed=on  enable_output=off  hold_output=off
  Frame Conversion1 : FrameConversion  OutFrame=Sample-based
  Sum of Elements1 : Sum  Inputs=+  OutDataType=sfix(16)  OutScaling=2^-10
  Out1 : Outport  OutDataType=sfix(16)  OutScaling=2^0
  wires:
  Delay Line1/1 -> Sum of Elements1/1
  Sum of Elements1/1 -> Frame Conversion1/1
  In1/1 -> Delay Line1/1
  Frame Conversion1/1 -> Out1/1

== system commtimrecresample/Timing Error Detector and Loop Filter (4 samples per symbol)/Timing Error Detector/Timing Error/Moving Average (0 initial conditions) ==
  In1 : Inport  OutDataType=sfix(16)  OutScaling=2^0
  Delay Line : dspbuff3/Delay Line  siz=50  ic=0  directfeed=on  enable_output=off  hold_output=off
  Frame Conversion : FrameConversion  OutFrame=Sample-based
  Sum of Elements : Sum  Inputs=+  OutDataType=sfix(16)  OutScaling=2^-10
  Out1 : Outport  OutDataType=sfix(16)  OutScaling=2^0
  wires:
  Delay Line/1 -> Sum of Elements/1
  Sum of Elements/1 -> Frame Conversion/1
  In1/1 -> Delay Line/1
  Frame Conversion/1 -> Out1/1

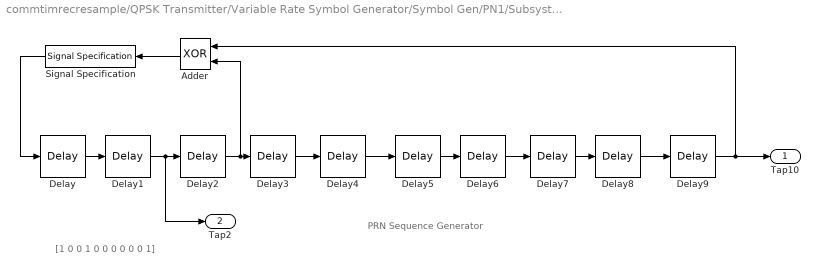
== system commtimrecresample/QPSK Transmitter/Variable Rate Symbol Generator/Symbol Gen/PN1/Subsystem ==
  note: [1 0 0 1 0 0 0 0 0 0 1]
  note: PRN Sequence Generator
  Adder : Logic  Orientation=left  Operator=XOR
  Delay{,3..8} (7 alike) : dspsigops/Delay  dly_unit=Samples  delay=1  ic_detail=on  dif_ic_for_ch=off  dif_ic_for_dly=off  ic=1  reset_popup=None
  Delay1 : dspsigops/Delay  dly_unit=Samples  delay=1  ic_detail=on  dif_ic_for_ch=off  dif_ic_for_dly=off  ic=0  reset_popup=None
  Delay2 : dspsigops/Delay  dly_unit=Samples  delay=1  ic_detail=on  dif_ic_for_ch=off  dif_ic_for_dly=off  ic=0  reset_popup=None
  Delay9 : dspsigops/Delay  dly_unit=Samples  delay=1  ic_detail=on  dif_ic_for_ch=off  dif_ic_for_dly=off  ic=0  reset_popup=None
  Signal Specification : SignalSpecification  Orientation=left  OutDataType=sfix(16)  OutScaling=2^0
  Tap10 : Outport  OutDataType=sfix(16)  OutScaling=2^0  InitialOutput=0
  Tap2 : Outport  Port=2  OutDataType=sfix(16)  OutScaling=2^0  InitialOutput=0
  wires:
  Delay2/1 -> Adder/2, Delay3/1
  Adder/1 -> Signal Specification/1
  Delay8/1 -> Delay9/1
  Delay7/1 -> Delay8/1
  Delay6/1 -> Delay7/1
  Delay5/1 -> Delay6/1
  Delay4/1 -> Delay5/1
  Delay3/1 -> Delay4/1
  Delay1/1 -> Tap2/1, Delay2/1
  Delay/1 -> Delay1/1
  Delay9/1 -> Tap10/1, Adder/1
  Signal Specification/1 -> Delay/1

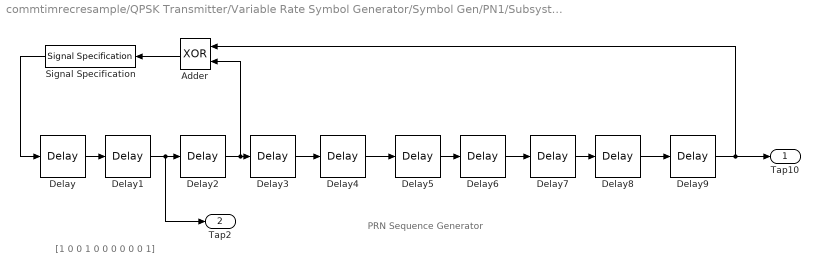
== system commtimrecresample/QPSK Transmitter/Variable Rate Symbol Generator/Symbol Gen/PN1/Subsystem1 ==
  note: PRN Sequence Generator
  note: [1 0 0 1 0 0 0 0 0 0 1]
  Adder : Logic  Orientation=left  Operator=XOR
  Delay{,1..5} (6 alike) : dspsigops/Delay  dly_unit=Samples  delay=1  ic_detail=on  dif_ic_for_ch=off  dif_ic_for_dly=off  ic=1  reset_popup=None
  Delay{6..9} (4 alike) : dspsigops/Delay  dly_unit=Samples  delay=1  ic_detail=on  dif_ic_for_ch=off  dif_ic_for_dly=off  ic=0  reset_popup=None
  Signal Specification : SignalSpecification  Orientation=left  OutDataType=sfix(16)  OutScaling=2^0
  Tap10 : Outport  OutDataType=sfix(16)  OutScaling=2^0  InitialOutput=0
  Tap2 : Outport  Port=2  OutDataType=sfix(16)  OutScaling=2^0  InitialOutput=0
  wires:
  Signal Specification/1 -> Delay/1
  Delay9/1 -> Adder/1, Tap10/1
  Delay/1 -> Delay1/1
  Delay1/1 -> Delay2/1, Tap2/1
  Delay3/1 -> Delay4/1
  Delay4/1 -> Delay5/1
  Delay5/1 -> Delay6/1
  Delay6/1 -> Delay7/1
  Delay7/1 -> Delay8/1
  Delay8/1 -> Delay9/1
  Adder/1 -> Signal Specification/1
  Delay2/1 -> Delay3/1, Adder/2

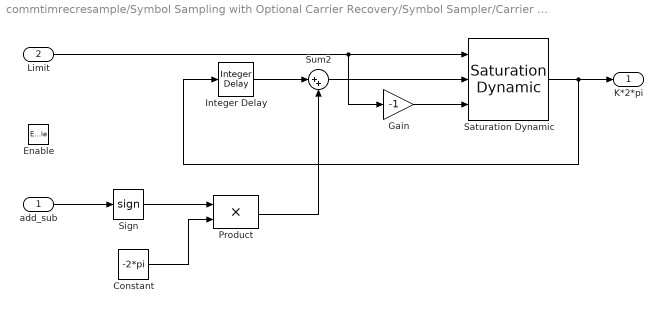
== system commtimrecresample/Symbol Sampling with Optional Carrier Recovery/Symbol Sampler/Carrier Recovery/Limited Phase Unwrapper/N*2*pi accumulator ==
  add_sub : Inport  OutDataType=sfix(16)  OutScaling=2^0
  Limit : Inport  Port=2  OutDataType=sfix(16)  OutScaling=2^0
  Enable : EnablePort
  Constant : Constant  Value=-2*pi  VectorParams1D=off  OutDataType=sfix(16)  OutScaling=2^0
  Gain : Gain  Gain=-1  ParameterDataType=sfix(16)  ParameterScaling=2^0  OutDataType=sfix(16)  OutScaling=2^0
  Integer Delay : simulink/Discrete/Integer Delay  vinit=0.0  samptime=-1  NumDelays=1
  Product : Product  OutDataType=sfix(16)  OutScaling=2^0  SaturateOnIntegerOverflow=on  OutDataTypeStr=Inherit: Same as first input
  Saturation Dynamic : simulink/Discontinuities/Saturation Dynamic  SystemSampleTime=-1  OutMin=[]  OutMax=[]  OutDataTypeStr=Inherit: Same as second input  OutDataType=sfix(16)  OutScaling=2^-10  DoSatur=off
  Sign : Signum
  Sum2 : Sum  Inputs=|++  OutDataType=sfix(16)  OutScaling=2^0  SaturateOnIntegerOverflow=on
  K*2*pi : Outport  OutDataType=sfix(16)  OutScaling=2^0
  wires:
  Integer Delay/1 -> Sum2/1
  Constant/1 -> Product/2
  Sign/1 -> Product/1
  Product/1 -> Sum2/2
  add_sub/1 -> Sign/1
  Sum2/1 -> Saturation Dynamic/2
  Saturation Dynamic/1 -> K*2*pi/1, Integer Delay/1
  Gain/1 -> Saturation Dynamic/3
  Limit/1 -> Gain/1, Saturation Dynamic/1

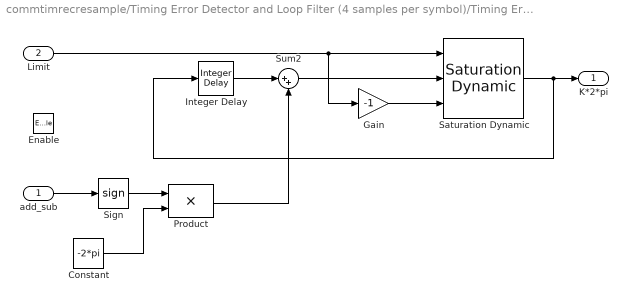
== system commtimrecresample/Timing Error Detector and Loop Filter (4 samples per symbol)/Timing Error Detector/Timing Error/Limited Phase Unwrapper/N*2*pi accumulator ==
  add_sub : Inport  OutDataType=sfix(16)  OutScaling=2^0
  Limit : Inport  Port=2  OutDataType=sfix(16)  OutScaling=2^0
  Enable : EnablePort
  Constant : Constant  Value=-2*pi  VectorParams1D=off  OutDataType=sfix(16)  OutScaling=2^0
  Gain : Gain  Gain=-1  ParameterDataType=sfix(16)  ParameterScaling=2^0  OutDataType=sfix(16)  OutScaling=2^0
  Integer Delay : simulink/Discrete/Integer Delay  vinit=0.0  samptime=-1  NumDelays=1
  Product : Product  OutDataType=sfix(16)  OutScaling=2^0  SaturateOnIntegerOverflow=on  OutDataTypeStr=Inherit: Same as first input
  Saturation Dynamic : simulink/Discontinuities/Saturation Dynamic  SystemSampleTime=-1  OutMin=[]  OutMax=[]  OutDataTypeStr=Inherit: Same as second input  OutDataType=sfix(16)  OutScaling=2^-10  DoSatur=off
  Sign : Signum
  Sum2 : Sum  Inputs=|++  OutDataType=sfix(16)  OutScaling=2^0  SaturateOnIntegerOverflow=on
  K*2*pi : Outport  OutDataType=sfix(16)  OutScaling=2^0
  wires:
  Integer Delay/1 -> Sum2/1
  Constant/1 -> Product/2
  Sign/1 -> Product/1
  Product/1 -> Sum2/2
  add_sub/1 -> Sign/1
  Sum2/1 -> Saturation Dynamic/2
  Saturation Dynamic/1 -> K*2*pi/1, Integer Delay/1
  Gain/1 -> Saturation Dynamic/3
  Limit/1 -> Gain/1, Saturation Dynamic/1
